simulink model "primer_2_8"  (R2018a)
settings: Solver=VariableStepAuto  StartTime=0.0  StopTime=10.0  RelTol=1e-3
settings Model: Creator=Teodor  LastModifiedBy=Teodor

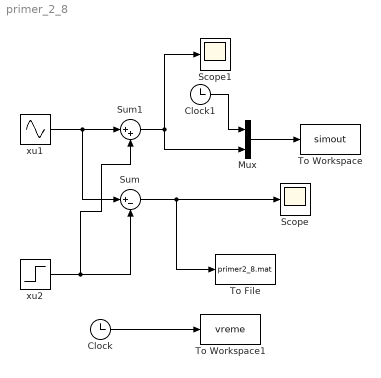
== system primer_2_8 ==
  Clock : Clock
  Clock1 : Clock
  Mux : Mux  Inputs=2
  Scope : Scope
  Scope1 : Scope
  Sum : Sum  Inputs=|+-
  Sum1 : Sum  Inputs=|++
  To File : ToFile  Filename=primer2_8.mat  MatrixName=izlaz
  To Workspace : ToWorkspace  VariableName=simout  SampleTime=-1
  To Workspace1 : ToWorkspace  VariableName=vreme  SampleTime=-1
  "xu1 " : Sin  SampleTime=0
  "xu2 " : Step  After=2  SampleTime=0
  wires:
  "xu1 "/1 -> Sum/1, Sum1/1
  "xu2 "/1 -> Sum1/2, Sum/2
  Sum/1 -> To File/1, Scope/1
  Sum1/1 -> Mux/2, Scope1/1
  Clock/1 -> To Workspace1/1
  Mux/1 -> To Workspace/1
  Clock1/1 -> Mux/1
